simulink model "Model"  (R2020b)
settings: Solver=VariableStepAuto  StartTime=0.0  StopTime=10000.0  RelTol=1e-3
undefined symbols (not defined in the file): a
settings Model: Creator=Nic  LastModifiedBy=Nic

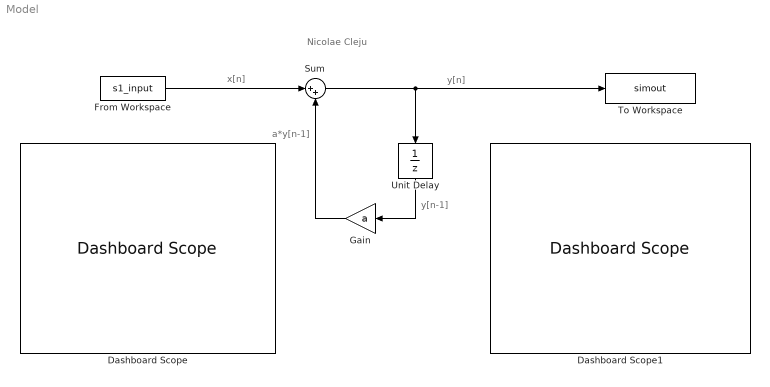
== system Model ==
  note: Nicolae Cleju
  note: a*y[n-1]
  note: y[n-1]
  note: x[n]
  note: y[n]
  Dashboard Scope : DashboardScope
  Dashboard Scope1 : DashboardScope
  From Workspace : FromWorkspace  VariableName=s1_input  SampleTime=1
  Gain : Gain  Gain=a
  Sum : Sum  Inputs=|++
  To Workspace : ToWorkspace  VariableName=simout  SampleTime=-1
  Unit Delay : UnitDelay  SampleTime=-1  HasFrameUpgradeWarning=on
  wires:
  From Workspace/1 -> Sum/1
  Sum/1 -> To Workspace/1, Unit Delay/1
  Unit Delay/1 -> Gain/1
  Gain/1 -> Sum/2
